simulink model "dip_student_sim_simulink"  (R2017a)
settings: Solver=ode45  StartTime=0.0  StopTime=10  FixedStep=0.01  MaxStep=0.05  RelTol=1e-3  EnableMultiTasking=on
settings Model: Creator=ut  LastModifiedBy=maam
settings DataIOCC: LimitDataPoints=on  SaveFormat=Array  SignalLoggingSaveFormat=ModelDataLogs
settings OptimizationCC: ExpressionDepthLimit=2147483647  InitFltsAndDblsToZero=on  LifeSpan=inf
settings DebuggingCC: SaveWithParameterizedLinksMsg=none  UnderspecifiedInitializationDetection=Classic  MergeDetectMultiDrivingBlocksExec=none  SignalResolutionControl=TryResolveAllWithWarning  SolverPrmCheckMsg=warning  MultiTaskDSMMsg=warning  MultiTaskCondExecSysMsg=none  FcnCallInpInsideContextMsg=warning  StateNameClashWarn=warning  SFUnexpectedBacktrackingDiag=warning  SFNoUnconditionalDefaultTransitionDiag=warning  SFExecutionAtInitializationDiag=none
settings HardwareCC: ProdBitPerPointer=32  ProdBitPerSizeT=32  ProdBitPerPtrDiffT=32  ProdLargestAtomicFloat=None  ProdIntDivRoundTo=Undefined  ProdEndianess=Unspecified  ProdWordSize=32  ProdHWDeviceType=32-bit Generic
settings ModelReferenceCC: PropagateSignalLabelsOutOfModel=off
settings GRTTargetCC: TargetFcnLib=ansi_tfl_tmw.mat  TargetLangStandard=C89/C90 (ANSI)  CombineOutputUpdateFcns=off  GRTInterface=on
settings ConfigComp: CovMetricSettings=dw  CovSaveCumulativeToWorkspaceVar=on  CovSaveSingleToWorkspaceVar=on  CovExternalEMLEnable=off

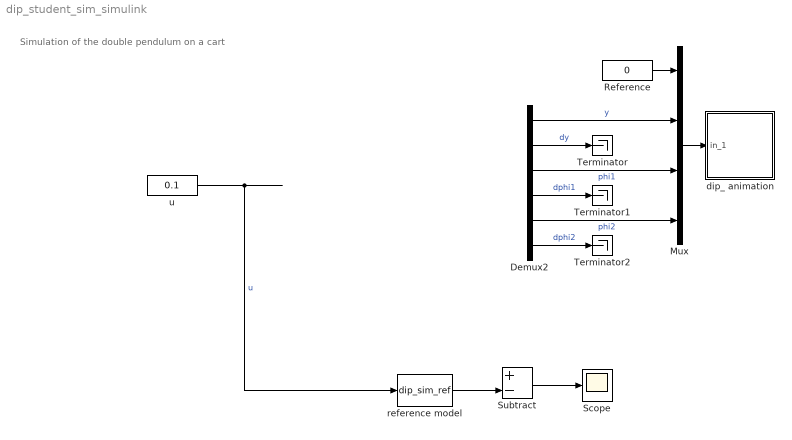
== system dip_student_sim_simulink ==
  note: Simulation of the double pendulum on a cart
  Demux2 : Demux  Outputs=6
  Mux : Mux
  Reference : Constant  Value=0
  Scope : Scope
  Subtract : Sum  Inputs=+-
  Terminator : Terminator
  Terminator1 : Terminator
  Terminator2 : Terminator
  dip_ animation : Subsystem  mask(Double Inverted Pendulum Plot){RefBlock=Reference}
      mask prompts: RefBlock "DC reference signal block name:"
      mask help: Double Inverted Pendulum Plot
      mask Help: Double Inverted Pendulum animation function using Handle graphics and S-function.
      mask Display: plot([-10 10],[0 0],[-2 -2 2 2],[0 1 1 0],[0 2],[1 3],[2 1],[3 5])
  reference model : M-S-Function  FunctionName=dip_sim_ref  Parameters=[0;0;0;0;0;0];
  u : Constant  Value=0.1
  wires:
  Mux/1 -> dip_ animation/1(in_1)
  Reference/1 -> Mux/1
  u/1 -> reference model/1  "u"
  ? -> Subtract/1, Demux2/1  "y"
  Demux2/1 -> Mux/2  "y"
  Demux2/3 -> Mux/3  "phi1"
  Demux2/5 -> Mux/4  "phi2"
  Demux2/2 -> Terminator/1  "dy"
  Demux2/4 -> Terminator1/1  "dphi1"
  Demux2/6 -> Terminator2/1  "dphi2"
  reference model/1 -> Subtract/2
  Subtract/1 -> Scope/1

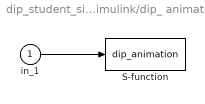
== system dip_student_sim_simulink/dip_ animation ==
  in_1 : Inport
  S-function : S-Function  FunctionName=dip_animation  Parameters=RefBlock  SFunctionDeploymentMode=off  EnableBusSupport=off
      settings: DeleteFcn=pendan([],[],[],'DeleteBlock');
  wires:
  in_1/1 -> S-function/1
